simulink model "Quadcopter"  (R2022a)
settings: Solver=VariableStepAuto  StartTime=0.0  StopTime=100  FixedStep=0.001  RelTol=1e-3
values from neighbouring files (symbols this model uses):
  airDensity = 1.2041    [Parameters.m]
  airframeCdx = 0.0    (= 0)    [Parameters.m]
  airframeDiameter = 0.33    [Parameters.m]
  airframeH = -0.016    [Parameters.m]
  airframeXY = 0.15    [Parameters.m]
  armLength = 0.23    [Parameters.m]
  commandToW2Gain = 27000    [Parameters.m]
  gravity = 9.81    [Parameters.m]
  motorMaxLimit = 100    [Parameters.m]
  motorMinLimit = 10    [Parameters.m]
  quadcopterMass = 1.4    [Parameters.m]
undefined symbols (not defined in the file or in its folder): diameter, dragCoeff, zTorqueConstant
libraries: aerolibasang x2, shared6dof x1, robotcorelib x1, dynamicsLibrary x1, sim3dlib x1, uavsim3dlib x1, aerolibanimutils x1
settings Model: Creator=fynnr  LastModifiedBy=fynnr

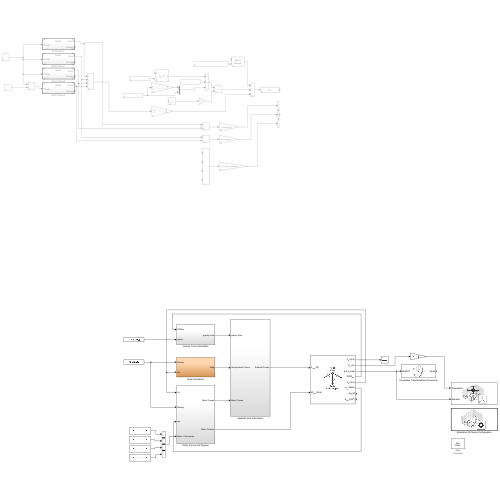
[thumbnail: Simulink's stored preview of the top-level diagram]
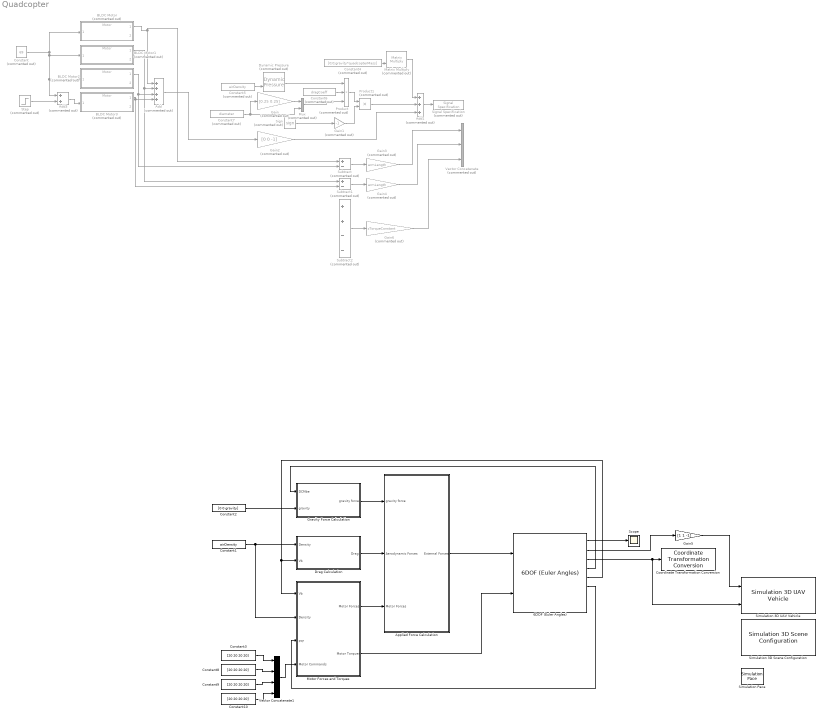
== system Quadcopter ==
  6DOF (Euler Angles) : shared6dof/6DOF (Euler Angles)  units=Metric (MKS)  mtype=Fixed  rep=Euler Angles  xme_0=[0 0 0]  Vm_0=[0 0 0]  eul_0=[0 0 0]  pm_0=[0 0 0]  mass_0=quadcopterMass  mass_e=0.5  mass_f=2.0  inertia=eye(3)  inertia_e=eye(3)  inertia_f=2*eye(3)  k_quat=1.0  vre_flag=on  abi_flag=off  aMode=0  xme_statename=''  Vm_statename=''  eul_statename=''  quat_statename=''  pm_statename=''  mass_statename=''
      settings: SourceProductBaseCode=AE,PW,DR,MT,VE
  Add : Sum  Commented=on  Inputs=++++
  Add1 : Sum  Commented=on  Inputs=+++
  Add3 : Sum  Commented=on
  Applied Force Calculation : Subsystem
  BLDC Motor{,1..3} (4 alike) : ModelReference  Commented=on  ModelNameDialog=Motor.slx  SimulationMode=Normal  ModelReferenceVersion=1.8
  Constant : Constant  Commented=on  Value=69
  Constant1 : Constant  Value=airDensity
  Constant{3,8..10} (4 alike) : Constant  Value=[20 20 20 20]
  Constant2 : Constant  Value=[0 0 gravity]
  Constant4 : Constant  Commented=on  Value=[0;0;gravity*quadcopterMass]
  Constant5 : Constant  Commented=on  Value=airDensity
  Constant6 : Constant  Commented=on  Value=dragCoeff
  Constant7 : Constant  Commented=on  Value=diameter
  Coordinate Transformation Conversion : robotcorelib/Coordinate Transformation Conversion  InputRepresentation=Euler Angles  InputEulerSequence=XYZ  ShowTrVecInputPort=on  OutputRepresentation=Quaternion  OutputEulerSequence=ZYX  ShowTrVecOutputPort=on  SimulateUsing=Interpreted execution
      settings: SourceProductBaseCode=RO,NV,RR,UV
  Drag Calculation : Subsystem
  Dynamic Pressure : aerolibasang/Dynamic Pressure  Commented=on
  Gain : Gain  Commented=on  Gain=[0.25 0.25]
  Gain1 : Gain  Commented=on  Gain=-1
  Gain2 : Gain  Commented=on  Gain=[0 0 -1]
  Gain3 : Gain  Commented=on  Gain=armLength
  Gain4 : Gain  Commented=on  Gain=armLength
  Gain5 : Gain  Gain=[1 1 -1]
  Gain6 : Gain  Commented=on  Gain=zTorqueConstant
  Gravity Force Calculation : Subsystem
  Matrix Multiply : Product  Commented=on  Multiplication=Matrix(*)
  Motor Forces and Torques : Subsystem
  Mux : Mux  Commented=on  Inputs=2
  Product : Product  Commented=on  Inputs=3
  Product1 : Product  Commented=on
  Scope : Scope
  Sign : Signum  Commented=on  ZeroCross=off
  Signal Specification : SignalSpecification  Commented=on  Dimensions=3
  Simulation 3D Scene Configuration : sim3dlib/Simulation 3D Scene Configuration  Priority=0  ProjectFormat=Default Scenes  SceneDesc=US city block  ProjectName=C:\Program Files\MATLAB\R2022a\toolbox\shared\sim3d_projects\automotive_project\UE4\WindowsNoEditor\VehicleSimulation.exe  ScenePath=/Game/Maps/USCityBlock  vehTagList={'Scene Origin';'SimulinkVehicle1'}  vehTag=SimulinkVehicle1  OpVisEn=off  Ts=1/60  EnableWindow=on  EnableRemoteAccess=off  EnableWeather=off  SunAltitude=40.0  SunAzimuth=90  clouds=10  wind=1  fog=0  rain=0  sensorTag=MainCamera1  sensorId=1  sensorName=MainCamera1  mountLoc=Origin  offsetFlag=off  tmountOffset=[0, 0, 0]  rmountOffset=[0, 0, 0]  HorizontalResolution=1280  VerticalResolution=720  HorizontalFOV=60  mountPoint=[0 0 0]  mountOrientation=[0 0 0]  aMode=4  ID=1
      settings: SourceProductBaseCode=VE,AE,DR,UV,VE
  Simulation 3D UAV Vehicle : uavsim3dlib/Simulation 3D UAV Vehicle  Priority=-1  Mesh=Quadrotor  MeshPath=/MathWorksUAVContent/UAVs/HexaRotorUAV/HexaRotor.HexaRotor  Color=Black  ActorName=SimulinkVehicle1  InitialTranslation=[0 0 0]  InitialRotation=[0 0 0]  SampleTime=-1  ActorType=SimulinkVehicle  ID=1  aMode=4  ActorTag=SimulinkVehicle1
      settings: SourceProductBaseCode=UV
  Simulation Pace : aerolibanimutils/Simulation Pace  SimulationPace=1  SleepMode=Auto  OutputPaceError=off  SampleTime=1/30
  Step : Step  Commented=on  After=0  SampleTime=0
  Subtract : Sum  Commented=on  Inputs=+-
  Subtract1 : Sum  Commented=on  Inputs=+-
  Subtract2 : Sum  Commented=on  Inputs=++--
  Vector Concatenate : Concatenate  Commented=on  NumInputs=3
  Vector Concatenate1 : Concatenate  NumInputs=4
  wires:
  6DOF (Euler Angles)/2 -> Gain5/1
  6DOF (Euler Angles)/1 -> Scope/1
  6DOF (Euler Angles)/3 -> Simulation 3D UAV Vehicle/2, Coordinate Transformation Conversion/1
  Gain5/1 -> Simulation 3D UAV Vehicle/1
  Applied Force Calculation/1(External Forces) -> 6DOF (Euler Angles)/1
  Motor Forces and Torques/1(Motor Forces) -> Applied Force Calculation/3(Motor Forces)
  Gravity Force Calculation/1(gravity force) -> Applied Force Calculation/1(gravity force)
  6DOF (Euler Angles)/4 -> Gravity Force Calculation/1(DCMbe)
  Motor Forces and Torques/2(Motor Torques) -> 6DOF (Euler Angles)/2
  Drag Calculation/1(Drag) -> Applied Force Calculation/2(Aerodynamic Forces)
  6DOF (Euler Angles)/5 -> Motor Forces and Torques/1(Vb), Drag Calculation/2(Vb)
  6DOF (Euler Angles)/6 -> Motor Forces and Torques/3(pqr)
  Constant1/1 -> Motor Forces and Torques/2(Density), Drag Calculation/1(Density)
  Subtract2/1 -> Gain6/1
  Step/1 -> Add3/2
  Gain4/1 -> Vector Concatenate/2
  Subtract1/1 -> Gain4/1
  BLDC Motor/1 -> Subtract/1, Add/1
  Add/1 -> Gain2/1
  Subtract/1 -> Gain3/1
  Add3/1 -> BLDC Motor3/1
  Product1/1 -> Add1/2
  Gain3/1 -> Vector Concatenate/1
  BLDC Motor3/1 -> Add/4, Subtract1/2
  Gain1/1 -> Product1/2
  Constant/1 -> BLDC Motor1/1, Add3/1, BLDC Motor2/1, BLDC Motor/1
  Mux/1 -> Product/3
  Gain2/1 -> Add1/3
  Constant7/1 -> Mux/2, Gain/1
  Gain/1 -> Mux/1
  Sign/1 -> Gain1/1
  BLDC Motor1/1 -> Subtract1/1, Add/2
  Product/1 -> Product1/1
  Constant6/1 -> Product/2
  Matrix Multiply/1 -> Add1/1
  Dynamic Pressure/1 -> Product/1
  Constant4/1 -> Matrix Multiply/2
  Constant5/1 -> Dynamic Pressure/2
  BLDC Motor2/1 -> Subtract/2, Add/3
  Gain6/1 -> Vector Concatenate/3
  Add1/1 -> Signal Specification/1
  Constant2/1 -> Gravity Force Calculation/2(gravity)
  Constant8/1 -> Vector Concatenate1/2
  Constant3/1 -> Vector Concatenate1/1
  Vector Concatenate1/1 -> Motor Forces and Torques/4(Motor Commands)
  Constant9/1 -> Vector Concatenate1/3
  Constant10/1 -> Vector Concatenate1/4

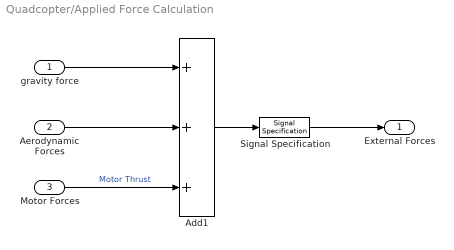
== system Quadcopter/Applied Force Calculation ==
  gravity force : Inport  Unit=N
  Aerodynamic Forces : Inport  Port=2  Unit=N
  Motor Forces : Inport  Port=3  Unit=N
  Add1 : Sum  Inputs=+++
  Signal Specification : SignalSpecification  Dimensions=3
  External Forces : Outport  Unit=N  VectorParamsAs1DForOutWhenUnconnected=off
  wires:
  Add1/1 -> Signal Specification/1
  Motor Forces/1 -> Add1/3  "Motor Thrust"
  Aerodynamic Forces/1 -> Add1/2
  gravity force/1 -> Add1/1
  Signal Specification/1 -> External Forces/1

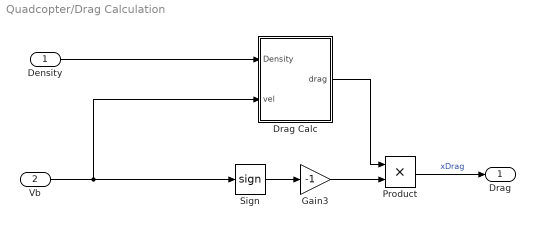
== system Quadcopter/Drag Calculation ==
  Density : Inport  Unit=kg/m^3
  Vb : Inport  Port=2  Unit=m/second
  Drag Calc : Subsystem
  Gain3 : Gain  Gain=-1
  Product : Product  RndMeth=Zero
  Sign : Signum  ZeroCross=off
  Drag : Outport  Unit=N  VectorParamsAs1DForOutWhenUnconnected=off
  wires:
  Density/1 -> Drag Calc/1(Density)
  Sign/1 -> Gain3/1
  Drag Calc/1(drag) -> Product/1
  Gain3/1 -> Product/2
  Product/1 -> Drag/1  "xDrag"
  Vb/1 -> Sign/1, Drag Calc/2(vel)

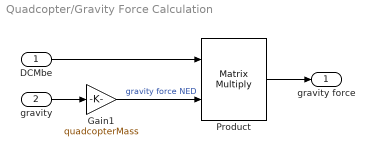
== system Quadcopter/Gravity Force Calculation ==
  DCMbe : Inport
  gravity : Inport  Port=2  Unit=m/s^2
  Gain1 : Gain  Gain=quadcopterMass
  Product : Product  Multiplication=Matrix(*)
  gravity force : Outport  Unit=N  VectorParamsAs1DForOutWhenUnconnected=off
  wires:
  gravity/1 -> Gain1/1
  Gain1/1 -> Product/2  "gravity force NED"
  Product/1 -> gravity force/1
  DCMbe/1 -> Product/1

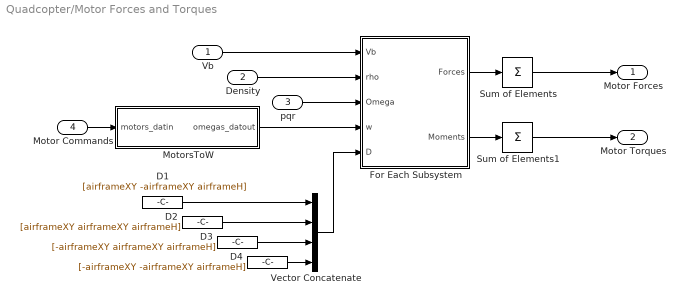
== system Quadcopter/Motor Forces and Torques ==
  Vb : Inport
  Density : Inport  Port=2
  pqr : Inport  Port=3
  Motor Commands : Inport  Port=4
  D1 : Constant  Value=[airframeXY -airframeXY airframeH]
  D2 : Constant  Value=[airframeXY airframeXY airframeH]
  D3 : Constant  Value=[-airframeXY airframeXY airframeH]
  D4 : Constant  Value=[-airframeXY -airframeXY airframeH]
  For Each Subsystem : Subsystem  TreatAsAtomicUnit=on
  MotorsToW : Subsystem
  Sum of Elements : Sum  Inputs=+  CollapseMode=Specified dimension  CollapseDim=2
  Sum of Elements1 : Sum  Inputs=+  CollapseMode=Specified dimension  CollapseDim=2
  Vector Concatenate : Concatenate  NumInputs=4  Mode=Multidimensional array  ConcatenateDimension=2
  Motor Forces : Outport  Unit=N  VectorParamsAs1DForOutWhenUnconnected=off
  Motor Torques : Outport  Port=2  Unit=N*m  VectorParamsAs1DForOutWhenUnconnected=off
  wires:
  D4/1 -> Vector Concatenate/4
  MotorsToW/1(omegas_datout) -> For Each Subsystem/4(w)
  Vector Concatenate/1 -> For Each Subsystem/5(D)
  For Each Subsystem/2(Moments) -> Sum of Elements1/1
  pqr/1 -> For Each Subsystem/3(Omega)
  Vb/1 -> For Each Subsystem/1(Vb)
  Motor Commands/1 -> MotorsToW/1(motors_datin)
  D1/1 -> Vector Concatenate/1
  D3/1 -> Vector Concatenate/3
  D2/1 -> Vector Concatenate/2
  Sum of Elements1/1 -> Motor Torques/1
  Density/1 -> For Each Subsystem/2(rho)
  Sum of Elements/1 -> Motor Forces/1
  For Each Subsystem/1(Forces) -> Sum of Elements/1

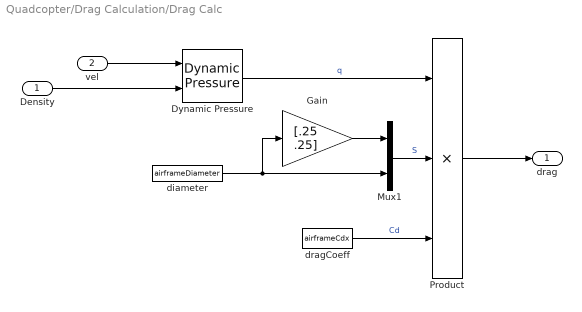
== system Quadcopter/Drag Calculation/Drag Calc ==
  Density : Inport  Unit=kg/m^3
  vel : Inport  Port=2  Unit=m/s
  Dynamic Pressure : aerolibasang/Dynamic Pressure
  Gain : Gain  Gain=[.25 .25]
  Mux1 : Mux  Inputs=2
  Product : Product  Inputs=3  RndMeth=Zero
  diameter : Constant  Value=airframeDiameter  SampleTime=0
  dragCoeff : Constant  Value=airframeCdx  SampleTime=0
  drag : Outport  Unit=N  VectorParamsAs1DForOutWhenUnconnected=off
  wires:
  Product/1 -> drag/1
  dragCoeff/1 -> Product/3  "Cd"
  Dynamic Pressure/1 -> Product/1  "q"
  diameter/1 -> Gain/1, Mux1/2
  Mux1/1 -> Product/2  "S"
  Gain/1 -> Mux1/1
  vel/1 -> Dynamic Pressure/1
  Density/1 -> Dynamic Pressure/2

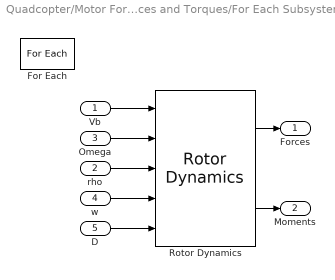
== system Quadcopter/Motor Forces and Torques/For Each Subsystem ==
  Vb : Inport  PortDimensions=3
  rho : Inport  Port=2  PortDimensions=1
  Omega : Inport  Port=3
  w : Inport  Port=4  Partition=on  PartitionDimension=2  PartitionWidth=1  PartitionOffset=0
  D : Inport  Port=5  Partition=on  PartitionDimension=2  PartitionWidth=1  PartitionOffset=0
  For Each : ForEach  DisableCoverage=on
  Rotor Dynamics : dynamicsLibrary/Rotor Dynamics  SystemSampleTime=-1  VariantActivationTime=update diagram  Latency=0  AutoFrameSizeCalculation=off
  Forces : Outport  ConcatenationDimension=2  VectorParamsAs1DForOutWhenUnconnected=off
  Moments : Outport  Port=2  ConcatenationDimension=2  VectorParamsAs1DForOutWhenUnconnected=off
  wires:
  Rotor Dynamics/1 -> Forces/1
  Rotor Dynamics/2 -> Moments/1
  Vb/1 -> Rotor Dynamics/1
  Omega/1 -> Rotor Dynamics/2
  rho/1 -> Rotor Dynamics/3
  D/1 -> Rotor Dynamics/5
  w/1 -> Rotor Dynamics/4

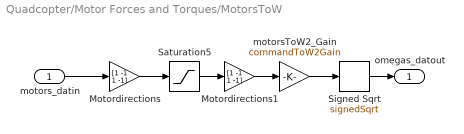
== system Quadcopter/Motor Forces and Torques/MotorsToW ==
  motors_datin : Inport
  Motordirections : Gain  Gain=[1 -1 1 -1]  ParamDataTypeStr=single  OutDataTypeStr=Inherit: Inherit via back propagation  SaturateOnIntegerOverflow=on
  Motordirections1 : Gain  Gain=[1 -1 1 -1]  ParamDataTypeStr=single  OutDataTypeStr=Inherit: Inherit via back propagation  SaturateOnIntegerOverflow=on
  Saturation5 : Saturate  UpperLimit=motorMaxLimit  LowerLimit=motorMinLimit  OutDataTypeStr=Inherit: Inherit via back propagation
  Signed Sqrt : Sqrt  Operator=signedSqrt  OutDataTypeStr=Inherit: Inherit via back propagation
  motorsToW2_Gain : Gain  Gain=commandToW2Gain  ParamDataTypeStr=single  OutDataTypeStr=Inherit: Inherit via back propagation  SaturateOnIntegerOverflow=on
  omegas_datout : Outport  VectorParamsAs1DForOutWhenUnconnected=off
  wires:
  motorsToW2_Gain/1 -> Signed Sqrt/1
  Motordirections/1 -> Saturation5/1
  Saturation5/1 -> Motordirections1/1
  Motordirections1/1 -> motorsToW2_Gain/1
  Signed Sqrt/1 -> omegas_datout/1
  motors_datin/1 -> Motordirections/1
